simulink model "PSH_Coffee_SimulinkStateFlow_V1"  (R2018a)
settings: Solver=FixedStepAuto  StartTime=0.0  StopTime=100  FixedStep=0.01  RelTol=1e-3  EnableMultiTasking=on
settings Model: EnablePacing=on  PacingRate=0.500000  Creator=tunn  LastModifiedBy=tunn
settings SolverCC: AutoInsertRateTranBlk=on
settings OptimizationCC: LifeSpan=inf
settings DebuggingCC: SFUnexpectedBacktrackingDiag=warning  SFNoUnconditionalDefaultTransitionDiag=warning  SFExecutionAtInitializationDiag=none
settings CodeAppCC: StateflowObjectComments=on
settings GRTTargetCC: TargetLangStandard=C89/C90 (ANSI)
settings ConfigComp: CovMetricSettings=dw  CovHtmlReporting=on  CovSaveCumulativeToWorkspaceVar=on  CovSaveSingleToWorkspaceVar=on  CovShowResultsExplorer=off  CovExternalEMLEnable=off

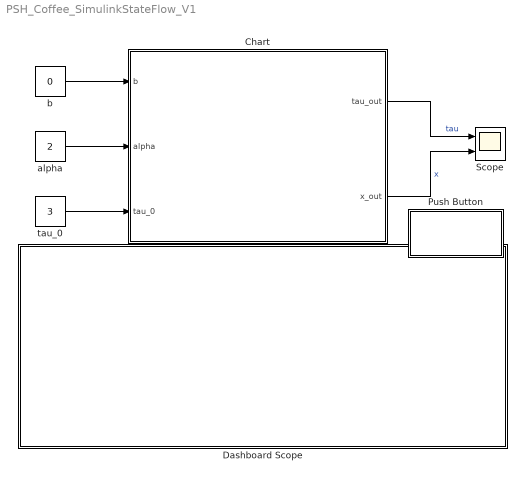
== system PSH_Coffee_SimulinkStateFlow_V1 ==
  Chart : Stateflow chart  TreatAsAtomicUnit=on
  Dashboard Scope : Subsystem  DialogController=hmiCreateDDGDialog  IsWebBlock=on  mask(MWDashboardBlock){webBlockId=0d24a4d6-6fd4-4889-9064-03b517be73d9, webBlockType=sdiscope, ShowInitialText=on, HMISrcModelName=PSH_Coffee_SimulinkStateFlow_V1}
      mask prompts: webBlockId "WebBlock Id"; webBlockType "WebBlock Type"; HMISrcModelName "Source Model"
      mask help: SimulinkHMI:dialogs:HMIScopeDialogDesc
      mask Help: helpview([docroot '/mapfiles/simulink.map'], 'hmi_scope')
      mask Display:
      | if strcmp(get_param(bdroot(gcb),'BlockDiagramType'), 'library')
      |     image([(matlabroot) '/toolbox/simulink/hmi/icons/DashboardScope.png']);
      | end
  Push Button : Subsystem  DialogController=hmiCreateDDGDialog  IsWebBlock=on  mask(MWDashboardBlock){webBlockId=8f9f16d7-94ec-48a8-890b-ffa68874c5a6, webBlockType=pushbutton, ShowInLibBrwoser=on, ShowInitialText=on, HMISrcModelName=PSH_Coffee_SimulinkStateFlow_V1}
      mask prompts: webBlockId "WebBlock Id"; webBlockType "WebBlock Type"; HMISrcModelName "Source Model"
      mask help: SimulinkHMI:dialogs:PushButtonDialogDesc
      mask Help: helpview([docroot '/mapfiles/simulink.map'], 'hmi_push_button')
      mask Display:
      | model = bdroot(gcb);
      | if strcmp(get_param(model,'BlockDiagramType'), 'library')
      |     image([(matlabroot) '/toolbox/simulink/hmi/icons/PushButton.png']);
      | end
  Scope : Scope  NumInputPorts=2
  alpha : Constant  Value=2
  b : Constant  Value=0
  tau_0 : Constant  Value=3
  wires:
  b/1 -> Chart/1(b)
  alpha/1 -> Chart/2(alpha)
  tau_0/1 -> Chart/3(tau_0)
  Chart/1(tau_out) -> Scope/1  "tau"
  Chart/2(x_out) -> Scope/2  "x"

== system PSH_Coffee_SimulinkStateFlow_V1/Dashboard Scope ==

== system PSH_Coffee_SimulinkStateFlow_V1/Push Button ==

== stateflow chart PSH_Coffee_SimulinkStateFlow_V1/Chart ==
  settings: updateMethod=CONTINUOUS
  state On
    du:
    x_dot    = -alpha ;
    tau_dot =  1        ;
    x_out    = x         ;
    tau_out = tau      ;
  state Off
    du:
    x_dot    = 0    ;
    tau_dot = 0    ;
    x_out    = x     ;
    tau_out = tau ;
  (default) -> Off : {
      | x    = 100 ;
      | tau = 0     ;
      | }
  Off -> On : [b]{tau = 0}
  On -> Off : [tau >= tau_0]
  data: b input; alpha input; tau_0 input; x local; tau_out output; x_out output; tau local
  data x settings: updateMethod=SF_CONTINUOUS_TIME_DATA
  data tau settings: updateMethod=SF_CONTINUOUS_TIME_DATA
